simulink model "mass_spring_damper"  (R2024a)
settings: Solver=VariableStepAuto  StartTime=0.0  StopTime=30  MaxStep=0.001  RelTol=1e-3
settings Model: Creator=varun  LastModifiedBy=varun

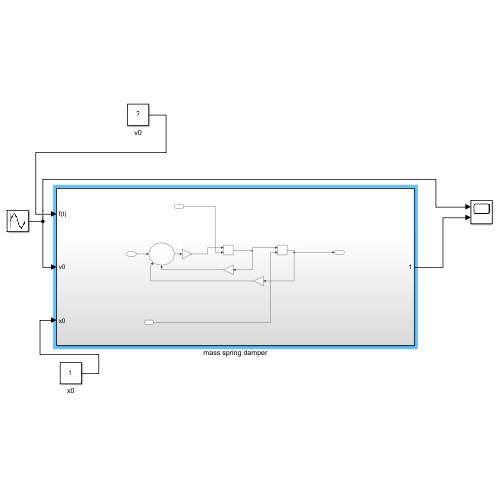
[thumbnail: Simulink's stored preview of the top-level diagram]
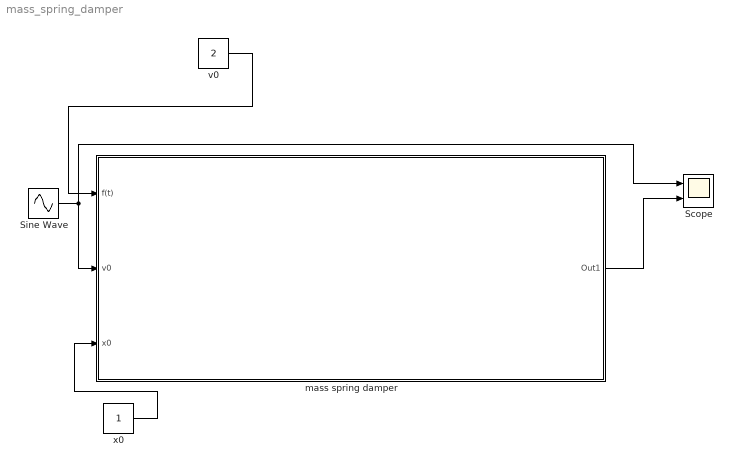
== system mass_spring_damper ==
  Scope : Scope  NumInputPorts=2
  Sine Wave : Sin  Amplitude=2  Frequency=2  SampleTime=0
  mass spring damper : Subsystem
  v0 : Constant  Value=2
  x0 : Constant
  wires:
  Sine Wave/1 -> mass spring damper/2(v0), Scope/1
  v0/1 -> mass spring damper/1(f(t))
  x0/1 -> mass spring damper/3(x0)
  mass spring damper/1(Out1) -> Scope/2

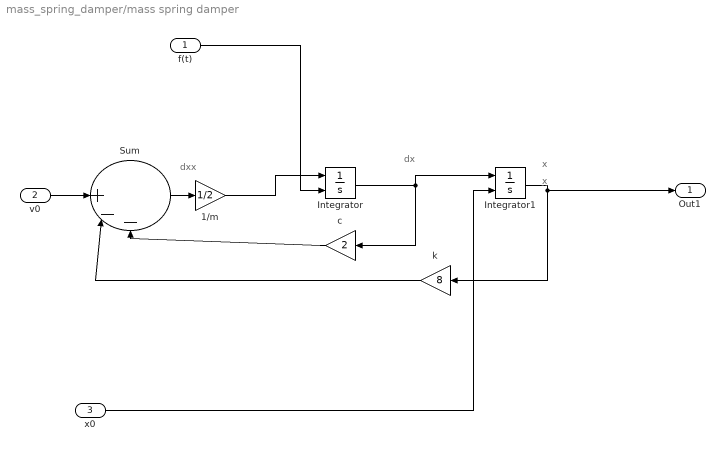
== system mass_spring_damper/mass spring damper ==
  note: x
  note: dx
  note: dxx
  note: x
  f(t) : Inport
  v0 : Inport  Port=2
  x0 : Inport  Port=3
  1/m : Gain  Gain=1/2
  Integrator : Integrator  InitialConditionSource=external  InitialCondition=2
  Integrator1 : Integrator  InitialConditionSource=external  InitialCondition=1
  Sum : Sum  Inputs=||+--
  c : Gain  Gain=2
  k : Gain  Gain=8
  Out1 : Outport
  wires:
  Integrator1/1 -> Out1/1, k/1
  1/m/1 -> Integrator/1
  Integrator/1 -> Integrator1/1, c/1
  k/1 -> Sum/2
  Sum/1 -> 1/m/1
  x0/1 -> Integrator1/2
  v0/1 -> Sum/1
  c/1 -> Sum/3
  f(t)/1 -> Integrator/2
